simulink model "LQG_NL"  (R2022b)
settings: Solver=VariableStepAuto  StartTime=0.0  StopTime=60  RelTol=1e-3
values from neighbouring files (symbols this model uses):
  A_tot = [A_nom B_nom*C_att ... (first row only)    [Inizializzazione_segway.m]    (also in LQG_controller.m = load("Matrici spazio di stato.mat","A_tot").A_tot; Matrici spazio di stato.mat = [0 79.8818966561 0 0 1 0 0 0 0 -0.384250591166 -200 0 ... (1)
  B_tot = [zeros(2,2); B_att]    [Inizializzazione_segway.m]    (also in LQG_controller.m = load("Matrici spazio di stato.mat","B_tot").B_tot; Matrici spazio di stato.mat = [0  0; 0  0; 894.427191  0; 0  894.427191])
  C_tot = [C_nom zeros(2,2)]    [Inizializzazione_segway.m]    (also in LQG_controller.m = load("Matrici spazio di stato.mat","C_tot").C_tot; Matrici spazio di stato.mat = [1  0  0  0; 0  1  0  0])
  D_tot = zeros(2,2)    [Inizializzazione_segway.m]    (also in LQG_controller.m = load("Matrici spazio di stato.mat","D_tot").D_tot; Matrici spazio di stato.mat = [0  0; 0  0])
  K = -lqr(A_tot,B_tot,Qr,Rr)    [LQG_controller.m]
  Km = 1.08    [Inizializzazione_segway.m]
  Qk = 0.01*diag([1 1])    [LQG_controller.m]
  Rk = (0.035)^2*diag([1 1])    [LQG_controller.m]
  Tm = 0.005    [Inizializzazione_segway.m]
undefined symbols (not defined in the file or in its folder): Continuous, Time
libraries: simulink x4, ctrlSharedLib x1
settings Model: Creator=mircocalzaretta  LastModifiedBy=mircocalzaretta

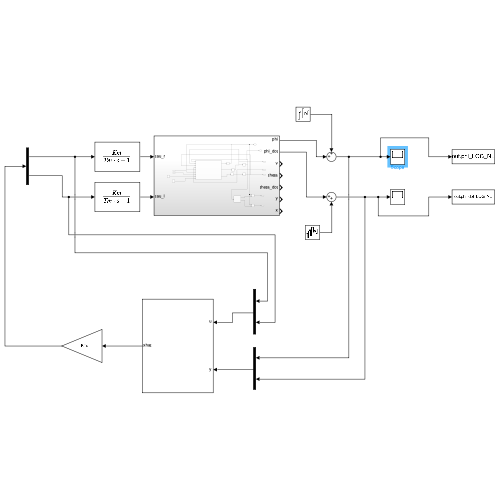
[thumbnail: Simulink's stored preview of the top-level diagram]
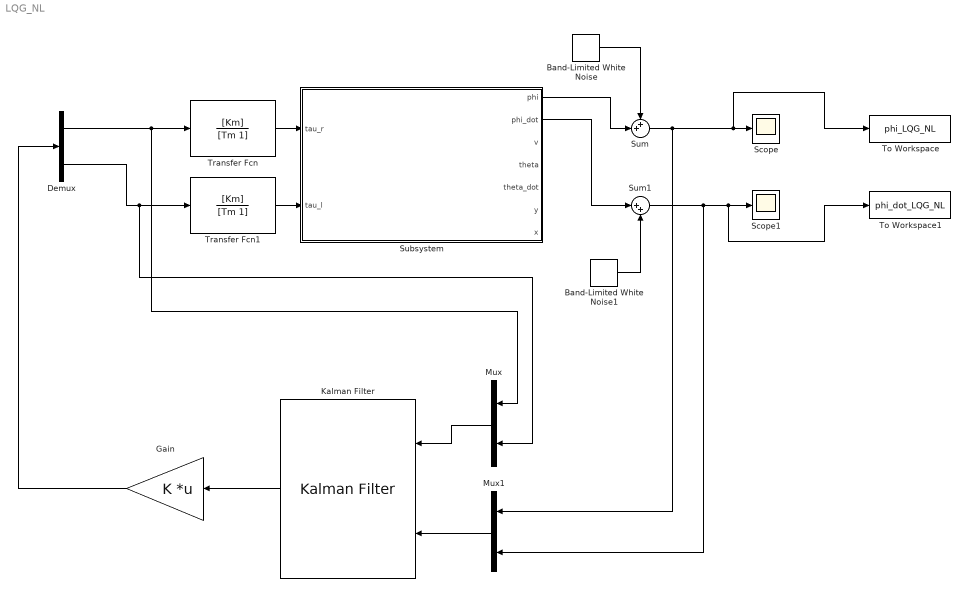
== system LQG_NL ==
  Band-Limited White Noise : simulink/Sources/Band-Limited White Noise  Cov=[Rk(1,1)]  Ts=0.01  seed=[23341]
  Band-Limited White Noise1 : simulink/Sources/Band-Limited White Noise  Cov=[Rk(2,2)]  Ts=0.01  seed=[23341]
  Demux : Demux  Outputs=2
  Gain : Gain  Gain=K  Multiplication=Matrix(K*u)
  Kalman Filter : ctrlSharedLib/Kalman Filter  TimeDomain=Continuous-Time  UseCurrentEstimator=on  ModelSource=Individual A, B, C, D matrices  ModelSourceVariable=ss(0.95,1,1,0,1)  A=A_tot  B=B_tot  C=C_tot  D=D_tot  NumberOfStates=1  NumberOfInputs=1  NumberOfOutputs=1  InitialEstimateSource=Dialog  X0=zeros(1,4)  P0=10  UseK=off  UseGH=on  NumberOfProcessNoiseInputs=1  G=B_tot  TimeInvariantG=on  H=0  TimeInvariantH=on  Q=Qk  TimeInvariantQ=on  R=Rk  TimeInvariantR=on  N=zeros(2,2)  TimeInvariantN=on  AddInputPort=on  AddEnablePort=off  OutputEstimatedY=off  OutputP=off  Ts=-1
  Mux : Mux  Inputs=2
  Mux1 : Mux  Inputs=2
  Scope : Scope
  Scope1 : Scope
  Subsystem : Subsystem
  Sum : Sum  Inputs=++|
  Sum1 : Sum  Inputs=|++
  To Workspace : ToWorkspace  VariableName=phi_LQG_NL  SaveFormat=Timeseries  SampleTime=-1
  To Workspace1 : ToWorkspace  VariableName=phi_dot_LQG_NL  SaveFormat=Timeseries  SampleTime=-1
  Transfer Fcn : TransferFcn  Numerator=[Km]  Denominator=[Tm 1]
  Transfer Fcn1 : TransferFcn  Numerator=[Km]  Denominator=[Tm 1]
  wires:
  Mux1/1 -> Kalman Filter/2
  Mux/1 -> Kalman Filter/1
  Subsystem/2(phi_dot) -> Sum1/1
  Subsystem/1(phi) -> Sum/2
  Band-Limited White Noise/1 -> Sum/1
  Band-Limited White Noise1/1 -> Sum1/2
  Sum/1 -> To Workspace/1, Scope/1, Mux1/1
  Sum1/1 -> To Workspace1/1, Scope1/1, Mux1/2
  Kalman Filter/1 -> Gain/1
  Gain/1 -> Demux/1
  Transfer Fcn/1 -> Subsystem/1(tau_r)
  Transfer Fcn1/1 -> Subsystem/2(tau_l)
  Demux/1 -> Mux/1, Transfer Fcn/1
  Demux/2 -> Mux/2, Transfer Fcn1/1

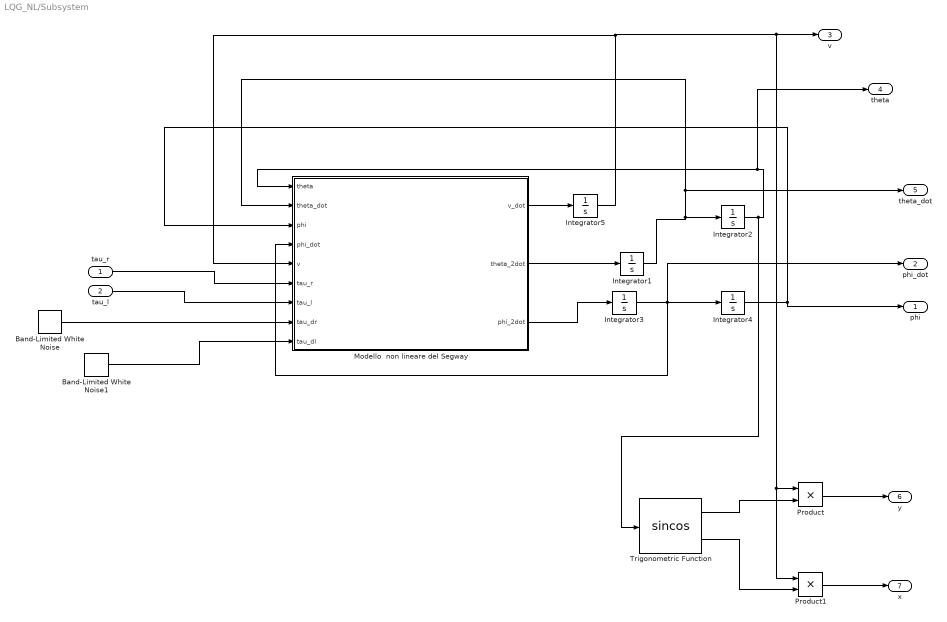
== system LQG_NL/Subsystem ==
  tau_r : Inport
  tau_l : Inport  Port=2
  Band-Limited White Noise : simulink/Sources/Band-Limited White Noise  Cov=[Qk(1,1)]  Ts=0.01  seed=[23341]
  Band-Limited White Noise1 : simulink/Sources/Band-Limited White Noise  Cov=[Qk(2,2)]  Ts=0.01  seed=[23341]
  Integrator{1..5} (5 alike) : Integrator
  Modello  non lineare del Segway : MATLAB Function  TreatAsAtomicUnit=on
  Product : Product
  Product1 : Product
  Trigonometric Function : Trigonometry  Operator=sincos
  phi : Outport
  phi_dot : Outport  Port=2
  v : Outport  Port=3
  theta : Outport  Port=4
  theta_dot : Outport  Port=5
  y : Outport  Port=6
  x : Outport  Port=7
  wires:
  Modello  non lineare del Segway/2(theta_2dot) -> Integrator1/1
  Modello  non lineare del Segway/3(phi_2dot) -> Integrator3/1
  Integrator4/1 -> phi/1, Modello  non lineare del Segway/3(phi)
  tau_l/1 -> Modello  non lineare del Segway/7(tau_l)
  Integrator3/1 -> phi_dot/1, Modello  non lineare del Segway/4(phi_dot), Integrator4/1
  tau_r/1 -> Modello  non lineare del Segway/6(tau_r)
  Integrator2/1 -> Trigonometric Function/1, theta/1, Modello  non lineare del Segway/1(theta)
  Integrator1/1 -> Integrator2/1, theta_dot/1, Modello  non lineare del Segway/2(theta_dot)
  Band-Limited White Noise/1 -> Modello  non lineare del Segway/8(tau_dr)
  Band-Limited White Noise1/1 -> Modello  non lineare del Segway/9(tau_dl)
  Modello  non lineare del Segway/1(v_dot) -> Integrator5/1
  Integrator5/1 -> Product1/1, Product/1, v/1, Modello  non lineare del Segway/5(v)
  Trigonometric Function/1 -> Product/2
  Trigonometric Function/2 -> Product1/2
  Product/1 -> y/1
  Product1/1 -> x/1

== matlab function LQG_NL/Subsystem/Modello  non lineare del Segway ==
  data: v_dot output; theta input; theta_dot input; phi input; phi_dot input; v input; tau_r input; tau_l input; theta_2dot output; phi_2dot output; tau_dr input; tau_dl input
function [v_dot, theta_2dot, phi_2dot] = SegwayDynamics(theta, theta_dot, phi, ...
    phi_dot, v, tau_r, tau_l, tau_dr, tau_dl)
    
    g = 9.81;
    m = 1.22;
    r = 0.13;
    a = 0.496/2;
    L = 0.2924;
    g = 9.81;
    M = 54;

    M_vdot = 2*(3/2*m +0.5*M);
    M_theta2dot = 2*(3/2*m*a^2 + 1/6*M*a^2 + 1/2*M*L^2*sin(phi)^2);
    M_phi2dot = 2*(1/2*m*r^2 + 2/3*M*L^2);
    M_vdot_phi2dot = -m*r+M*L*cos(phi);
    c_v = -M*L*sin(phi)*(theta_dot^2 + phi_dot^2);
    c_thetadot = 2*M*L^2*sin(phi)*cos(phi)*theta_dot*phi_dot+M*L*sin(phi)...
                    *v*theta_dot;
    c_phidot = -M*L^2*sin(phi)*cos(phi)*theta_dot^2;
    g_phidot = -M*L*g*sin(phi);
    
    I = [M_vdot 0 M_vdot_phi2dot;
         0 M_theta2dot 0;
         M_vdot_phi2dot 0 M_phi2dot];
    
    C = [c_v c_thetadot c_phidot]';
    G = [0 0 g_phidot]';
    
    Ing = [1/r 1/r;
           a/r -a/r;
           -1 -1];

    csi567_dot = inv(I)*(Ing*[tau_r + tau_dr,tau_l + tau_dl]' - C -G);
    v_dot = csi567_dot(1);
    theta_2dot = csi567_dot(2);
    phi_2dot = csi567_dot(3);
